simulink model "Thermal_model"  (R2021a)
settings: Solver=VariableStepAuto  StartTime=0.0  StopTime=48  RelTol=1e-3
values from neighbouring files (symbols this model uses):
  C = 1005.4    [Thermal_modeling_house_parameters.m]
  cost = 2.5/(3.6*10^6)    (= 6.94444444444e-07)    [Thermal_modeling_house_parameters.m]
  M = 5987.7684    [Thermal_modeling_house_parameters.m]
  Mdot = 3600    [Thermal_modeling_house_parameters.m]
  Req = 0.0000004    (= 4e-07)    [Thermal_modeling_house_parameters.m]
  Theater = 50    [Thermal_modeling_house_parameters.m]
settings Model: Creator=mluser  LastModifiedBy=mluser

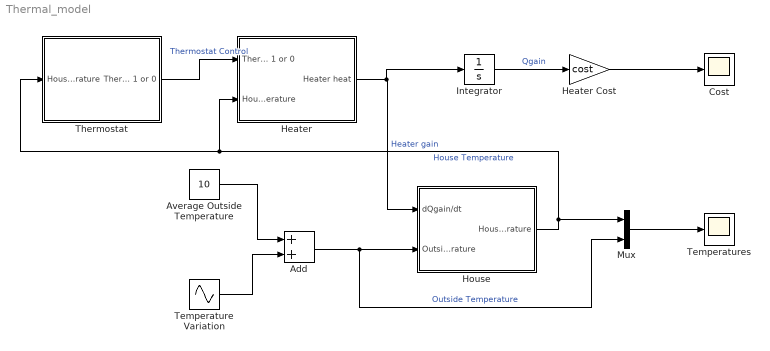
== system Thermal_model ==
  Add : Sum
  Average Outside Temperature : Constant  Value=10
  Cost : Scope
  Heater : Subsystem
  Heater Cost : Gain  Gain=cost
  House : Subsystem
  Integrator : Integrator
  Mux : Mux  Inputs=2
  Temperature Variation : Sin  Amplitude=5  Frequency=2*pi/24  SampleTime=0
  Temperatures : Scope
  "Thermostat\t" : Subsystem
  wires:
  Average Outside Temperature/1 -> Add/1
  Temperature Variation/1 -> Add/2
  Heater/1(Heater heat) -> Integrator/1, House/1(dQgain/dt)  "Heater gain"
  Add/1 -> Mux/2, House/2(Outside temperature)  "Outside Temperature"
  House/1(House temperature) -> Mux/1, Heater/2(House Temperature), "Thermostat\t"/1(House Temperature)  "House Temperature"
  "Thermostat\t"/1(Thermostat control ON or OFF 1 or 0) -> Heater/1("Thermostat Control ON or OFF 1 or 0 ")  "Thermostat Control"
  Integrator/1 -> Heater Cost/1  "Qgain"
  Heater Cost/1 -> Cost/1
  Mux/1 -> Temperatures/1

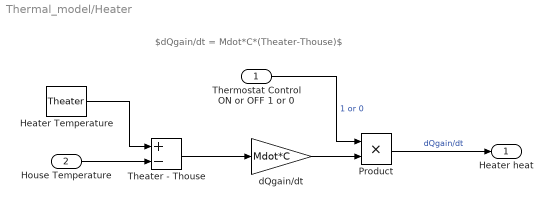
== system Thermal_model/Heater ==
  note: $dQgain/dt = Mdot*C*(Theater-Thouse)$
  "Thermostat Control ON or OFF 1 or 0 " : Inport
  House Temperature : Inport  Port=2
  Heater Temperature : Constant  Value=Theater
  Product : Product
  Theater - Thouse : Sum  Inputs=+-
  dQgain/dt : Gain  Gain=Mdot*C
  Heater heat : Outport
  wires:
  Heater Temperature/1 -> Theater - Thouse/1
  House Temperature/1 -> Theater - Thouse/2
  Theater - Thouse/1 -> dQgain/dt/1
  "Thermostat Control ON or OFF 1 or 0 "/1 -> Product/1  "1 or 0"
  Product/1 -> Heater heat/1  "dQgain/dt"
  dQgain/dt/1 -> Product/2

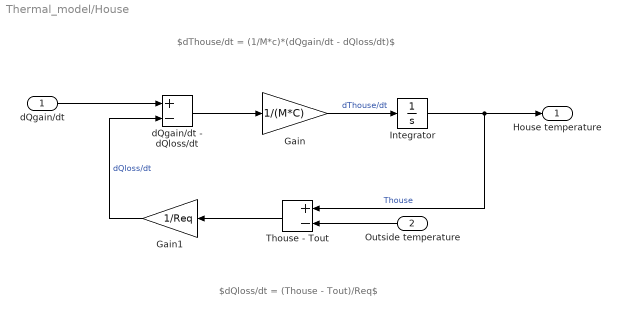
== system Thermal_model/House ==
  note: $dQloss/dt = (Thouse - Tout)/Req$
  note: $dThouse/dt = (1/M*c)*(dQgain/dt - dQloss/dt)$
  dQgain/dt : Inport
  Outside temperature : Inport  Port=2
  Gain : Gain  Gain=1/(M*C)
  Gain1 : Gain  Gain=1/Req
  Integrator : Integrator
  Thouse - Tout : Sum  Inputs=+-
  dQgain/dt - dQloss/dt : Sum  Inputs=+-
  House temperature : Outport
  wires:
  dQgain/dt/1 -> dQgain/dt - dQloss/dt/1
  dQgain/dt - dQloss/dt/1 -> Gain/1
  Gain/1 -> Integrator/1  "dThouse/dt"
  Integrator/1 -> Thouse - Tout/1, House temperature/1  "Thouse"
  Outside temperature/1 -> Thouse - Tout/2
  Thouse - Tout/1 -> Gain1/1
  Gain1/1 -> dQgain/dt - dQloss/dt/2  "dQloss/dt"

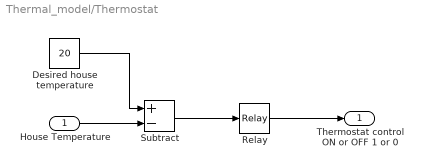
== system Thermal_model/Thermostat	 ==
  House Temperature : Inport
  Desired house temperature : Constant  Value=20
  Relay : Relay  OnSwitchValue=2  OffSwitchValue=-2
  Subtract : Sum  Inputs=+-
  Thermostat control ON or OFF 1 or 0 : Outport
  wires:
  Desired house temperature/1 -> Subtract/1
  House Temperature/1 -> Subtract/2
  Subtract/1 -> Relay/1
  Relay/1 -> Thermostat control ON or OFF 1 or 0/1
